simulink model "patient_covid"  (R2019b)
settings: Solver=FixedStepDiscrete  StartTime=0.0  StopTime=10.0  FixedStep=0.1  RelTol=1e-3  EnableMultiTasking=on
settings Model: EnablePacing=on  PacingRate=1.400000  Creator=Paul Guilot  LastModifiedBy=Paul Guilot
settings SolverCC: AutoInsertRateTranBlk=on
settings DataIOCC: LimitDataPoints=on
settings OptimizationCC: LifeSpan=inf
settings DebuggingCC: AllowSymbolicDim=off  SFUnexpectedBacktrackingDiag=warning  SFNoUnconditionalDefaultTransitionDiag=warning  SFExecutionAtInitializationDiag=none  ArithmeticOperatorsInVariantConditions=warning
settings SFSimCC: SimUseLocalCustomCode=off  CustomCodeUndefinedFunction=UseInterfaceOnly
settings RTWCC: RTWUseLocalCustomCode=off
settings CodeAppCC: StateflowObjectComments=on
settings GRTTargetCC: TargetLangStandard=C89/C90 (ANSI)  GeneratePreprocessorConditionals=Disable all
settings ConfigComp: CovMetricSettings=dw  CovHtmlReporting=on  CovSaveCumulativeToWorkspaceVar=on  CovSaveSingleToWorkspaceVar=on  CovShowResultsExplorer=off  CovExternalEMLEnable=off  CovSFcnEnable=off

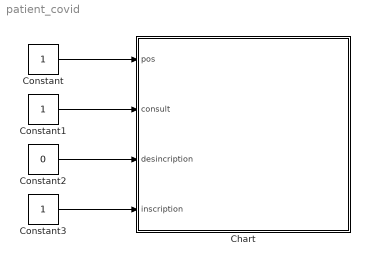
== system patient_covid ==
  Chart : Stateflow chart  TreatAsAtomicUnit=on
  Constant : Constant
  Constant1 : Constant
  Constant2 : Constant  Value=0
  Constant3 : Constant
  wires:
  Constant/1 -> Chart/1(pos)
  Constant1/1 -> Chart/2(consult)
  Constant2/1 -> Chart/3(desincription)
  Constant3/1 -> Chart/4(inscription)

== stateflow chart patient_covid/Chart ==
  state Consultation
  state Present
    exit: inscrit == 0
    state Test [parallel]
      during:
      if consult == 1
      if pos == 1
      test = 1
      end
      end
      settings: executionOrder=1
    state Suivi [parallel]
      settings: executionOrder=2
      settings: description=|
          | Suivi
          | Attribution d'un médecin au patient : son médecin traitant si celui-ci est sur la plateforme.
  state Absent
    inscrit = 0
    test = 0
  state Test
    during :
    if pos == 1
    test = 1
    else
    test = 0
    end
  Present -> Absent [order 3] : after(d, sec) [test == 0]
  Present -> Absent [order 2] : [ desincription == 1]
  Consultation -> Absent [order 2]
  (default) -> Absent
  Consultation -> Present [order 1] : [inscription== 1]{inscrit == 1}
  Absent -> Consultation [order 1] : [consult==1]
  Absent -> Test [order 2] : [consult == 0]
  Present -> Absent [order 1] : after(guerison, sec)
  Test -> Absent [order 2] : after(d, sec) [test == 0]
  Test -> Present [order 1] : after(d, sec)[test == 1]{inscrit == 1}
  data: d constant double =2; inscrit local; guerison constant double =5; pos input =1; consult input; desincription input; inscription input; test local
